simulink model "MPPI"  (R2021b)
settings: Solver=FixedStepAuto  StartTime=0.0  StopTime=10.0  FixedStep=0.01  RelTol=1e-3
undefined symbols (not defined in the file): gaosu, pathdata2
settings Model: Creator=huang.hj  LastModifiedBy=huang.hj

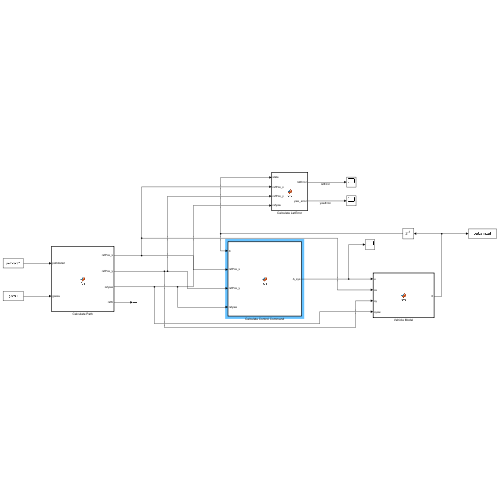
[thumbnail: Simulink's stored preview of the top-level diagram]
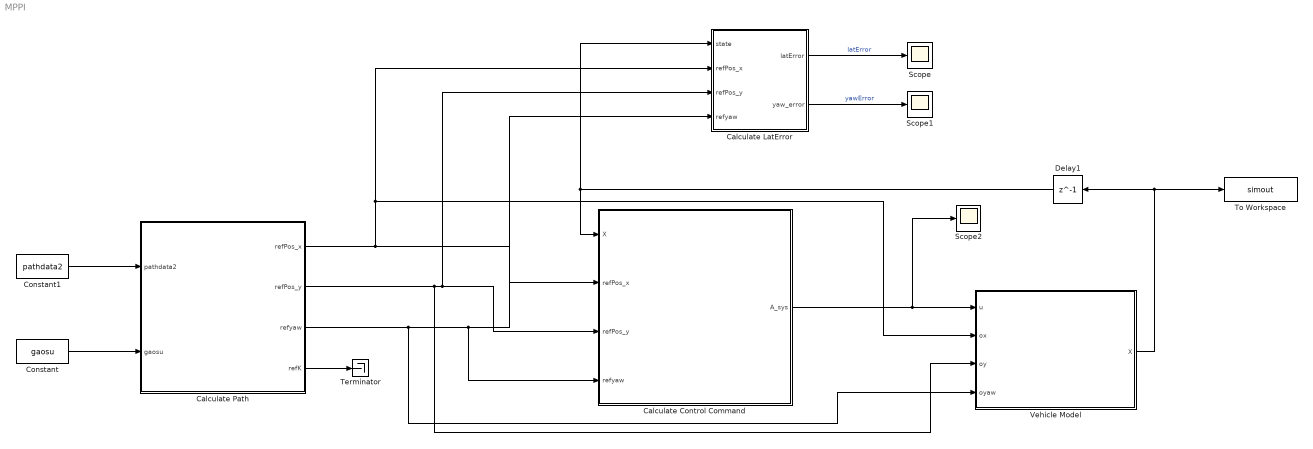
== system MPPI ==
  Calculate Control Command : MATLAB Function  TreatAsAtomicUnit=on
  Calculate LatError : MATLAB Function  TreatAsAtomicUnit=on
  Calculate Path : MATLAB Function  TreatAsAtomicUnit=on
  Constant : Constant  Value=gaosu
  Constant1 : Constant  Value=pathdata2
  Delay1 : Delay  DelayLength=1
  Scope : Scope
  Scope1 : Scope
  Scope2 : Scope
  Terminator : Terminator
  To Workspace : ToWorkspace  VariableName=simout  SaveFormat=Timeseries  SampleTime=-1
  Vehicle Model : MATLAB Function  TreatAsAtomicUnit=on
  wires:
  Constant1/1 -> Calculate Path/1(pathdata2)
  Constant/1 -> Calculate Path/2(gaosu)
  Calculate Path/4(refK) -> Terminator/1
  Calculate Path/3(refyaw) -> Vehicle Model/4(oyaw), Calculate Control Command/4(refyaw), Calculate LatError/4(refyaw)
  Calculate Path/2(refPos_y) -> Vehicle Model/3(oy), Calculate LatError/3(refPos_y), Calculate Control Command/3(refPos_y)
  Calculate Path/1(refPos_x) -> Vehicle Model/2(ox), Calculate LatError/2(refPos_x), Calculate Control Command/2(refPos_x)
  Calculate LatError/1(latError) -> Scope/1  "latError"
  Calculate LatError/2(yaw_error) -> Scope1/1  "yawError"
  Vehicle Model/1(X) -> Delay1/1, To Workspace/1
  Calculate Control Command/1(A_sys) -> Scope2/1, Vehicle Model/1(u)
  Delay1/1 -> Calculate Control Command/1(X), Calculate LatError/1(state)

== matlab function MPPI/Calculate LatError ==
  data: state input; latError output; refPos_x input; refPos_y input; refyaw input; yaw_error output
function [latError, yaw_error] = fcn(state, refPos_x,refPos_y, refyaw)
% persistent step last_latError last_yaw_error
%dt = 0.001;
x = state(1);
y = state(2);
yaw = state(3);
idx = calc_target_index(x,y, refPos_x,refPos_y);


% 求位置、航向角参考量
x_r = refPos_x(idx);
y_r = refPos_y(idx);
heading_r = refyaw(idx); 

% 求位置、航向角的误差
x_error  = x - x_r;
y_error = y - y_r;
yaw_error =  yaw - heading_r;

% 根据百度Apollo，计算横向误差
latError = y_error*cos(heading_r) - x_error*sin(heading_r);

% 将误差值赋值到状态量
% X(1,1) = x_error; 
% X(2,1) = y_error;  
% X(3,1) = yaw_error;

% if isempty(step)
%     latError_rate = 0;
%     yaw_error_rate = 0;
%     last_latError = 0;
%     
%     step = 1;
% else
%     latError_rate = (last_latError-latError)/dt;
%     yaw_error_rate = (last_yaw_error-yaw_error)/dt;
% % end
% last_yaw_error = yaw_error;
% last_latError = latError;
end

== matlab function MPPI/Vehicle Model ==
  data: u input; X output; ox input; oy input; oyaw input
function X = fcn(u,ox,oy,oyaw)
persistent last_state
v = 10;
if isempty(last_state)
    last_state = [ox(1);oy(1);oyaw(1)];
end
dt = 0.01;
L = 4;
xo = last_state(1);
yo = last_state(2);
yaw = last_state(3);
x = xo + v * cos(yaw) * dt;
y = yo + v * sin(yaw) * dt;
yaw = yaw + v / L * tan(u(1)) * dt;
X = [x;y;yaw];
last_state = X;
end

== matlab function MPPI/Calculate Control Command ==
  data: A_sys output; X input; refPos_x input; refPos_y input; refyaw input
function A_sys = fcn(X, refPos_x,refPos_y, refyaw)
persistent last_u u control_a
%% 相关参数定义
K = 200;
N = 50;
param.dt = 0.01;
param.v = 10;              %5m/s
param.m = 1400;
param.g = 9.81;
param.L = 4;


% Variance and Lamda
param.lambda = 10;
param.variance = 1;
param.R = 1;

param.Q = [30 0 0 0;
           0 0 0 0;
           0 0 70 0;
           0 0 0 0];

param.r = 1;
param.omega = 2; %2

filter_param.ts = param.dt;
filter_param.epsilon = 0.78;
filter_param.cutfreq = 4;


% Initialization of input for N time horizone
v = zeros(K,N-1);

% x_cur = zeros(3,N-1);
% u_opt = zeros(1,N-1);
% u_all = zeros(1,N-1,K);
% d_d_u = zeros(1,N-1,K);
if isempty(last_u)
    last_u = 0;
    u = zeros(1,N-1);
    control_a = zeros(1,N-1);
end
a = zeros(K,N-1);
Stk = zeros(1,K);
delta_u = zeros(K,N-1);
delta_limit = deg2rad(30);
d_delta_limit = deg2rad(200);
% Calculating cost for K samples and N finite horizone
for k = 1:K
    x = zeros(3,N);
    x(:,1) = X;
    d_d_u = normrnd(0,param.variance,[1, N-1]);
    %         u_all(:,:,k) = u + d_u;
    for j = 1:N-1
        %d_d_u(j) = clamp_u(d_d_u(j),d_delta_limit,-d_delta_limit);
        delta_u(k,j) = d_d_u(j);
        v(k,j) = u(j)+delta_u(k,j);
        v(k,j) = clamp_u(v(k,j),d_delta_limit,-d_delta_limit);
        %a(k,j) = control_a(j) + v(k,j)*param.dt;
        if j == 1
            a(k,j) = control_a(1) + v(k,j)*param.dt;
        else
            a(k,j) = a(k,j-1) + v(k,j)*param.dt;
        end
        %限制车辆转角极限值
        a(k,j) = clamp_u(a(k,j), delta_limit, -delta_limit);
        x(:,j+1) = vehicle_kinetics(x(:,j) ,a(k,j) ,param);
        [Cost ,~,~] = cost_func(x(:,j+1), a(k,j), refPos_x ,refPos_y ,refyaw ,param);
        Stk(k) = Stk(k) + Cost;
    end
    Stk(k) = Stk(k) + cost_action(a(k,:), last_u, param);
end
for n = 1:N-1
    u(n) = u(n) + totalEntropy(Stk(:) ,delta_u(:,n) ,param);
    control_a(n) = control_a(n) + u(n)*param.dt;
end

if control_a(1) > delta_limit
    A_sys = delta_limit;
elseif control_a(1) < -delta_limit
    A_sys = -delta_limit;
else
    A_sys = control_a(1);
end

A_sys = double_lowpass_filter(A_sys, filter_param);
last_u = A_sys;
u = [u(2:N-1) 0];
%a = [a(2:N-1) 0];
end


function filtered = double_lowpass_filter(unfilter, filter_param)
persistent p_output p_p_output

if isempty(p_output)
    p_output = 0;
    p_p_output = 0;
end

ts = filter_param.ts;
cutoff_freq = filter_param.cutfreq;
epsilon = filter_param.epsilon;

wn = 2*pi*cutoff_freq;

coeff_b1 = -2*exp(-epsilon*wn*ts)*cos(wn*ts*sqrt(1-epsilon^2));
coeff_b2 = exp(-2*wn*epsilon*ts);
coeff_a1 = 1+coeff_b1 + coeff_b2;

filtered = coeff_a1 * unfilter - coeff_b1 * p_output - coeff_b2 * p_p_output;

p_p_output = p_output;
p_output = filtered;
end

function [entropy] = totalEntropy(Sk , del_uk, param)
    % Calculation of expectency over trajectory 
    
    % Normalization of cost function 
%     Sk = Sk./sum(Sk);


    n = length(Sk);
    lambda = param.lambda;
    sum1 = 0;
    sum2 = 0;
    for i = 1:n
        sum1 = sum1 + exp(-(1/lambda)*Sk(i))*del_uk(i);
        sum2 = sum2 + exp(-(1/lambda)*Sk(i));
    end
    if sum2 == 0
        entropy = 0;
    else
        entropy = sum1/sum2;
    end
end

function cost = cost_action(a,a0,param)

omega = param.omega;

cost = (a(1)-a0)*omega*(a(1)-a0);
num = length(a);
for i = 2:num
    cost = cost + (a(i)-a(i-1))*omega*(a(i)-a(i-1));
end
end

function X = vehicle_kinetics(X ,delta ,param)
v = param.v;
dt = param.dt;
L = param.L;
xo = X(1);
yo = X(2);
yaw = X(3);
x = xo + v * cos(yaw) * dt;
y = yo + v * sin(yaw) * dt;
yaw = yaw + v / L * tan(delta) * dt;
X = [x;y;yaw];
end

function result = clamp_u(u, u_max, u_min)
result = u;
if result>u_max
    result = u_max;
end
if result<u_min
    result = u_min;
end
end

function [Cost ,idx,latError] = cost_func(state, u, refPos_x,refPos_y, refyaw, param)
persistent step last_latError last_yaw_error
dt = param.dt;
x = state(1);
y = state(2);
yaw = state(3);
%idx = calc_target_index(x,y, refPos_x,refPos_y);
idx = 1;

% 求位置、航向角参考量
x_r = refPos_x(idx);
y_r = refPos_y(idx);
heading_r = refyaw(idx); 

% 求位置、航向角的误差
x_error  = x - x_r;
y_error = y - y_r;
yaw_error =  yaw - heading_r;

% 根据百度Apollo，计算横向误差
latError = y_error*cos(heading_r) - x_error*sin(heading_r);

% 将误差值赋值到状态量
% X(1,1) = x_error; 
% X(2,1) = y_error;  
% X(3,1) = yaw_error;

if isempty(step)
    latError_rate = 0;
    yaw_error_rate = 0;
    last_latError = 0;
    last_yaw_error = 0;
    step = 1;
else
    latError_rate = (last_latError-latError)/dt;
    yaw_error_rate = (last_yaw_error-yaw_error)/dt;
end
X = zeros(4,1);
X(1,1) = latError; 
X(2,1) = latError_rate;  
X(3,1) = yaw_error;
X(4,1) = yaw_error_rate;
% Q1 = -5.127*exp(-36.37*abs(latError))+5.127*exp(0.7583*abs(latError));
% Q2 = -5.127*exp(-36.37*abs(latError)*dt)+5.127*exp(0.7583*abs(latError)*dt);
% Q3 = -5.127*exp(-36.37*abs(yaw_error))+5.127*exp(0.7583*abs(yaw_error));
% Q4 = -5.127*exp(-36.37*abs(yaw_error_rate*dt))+5.127*exp(0.7583*abs(yaw_error_rate*dt));
% Q = [Q1 0 0 0;
%      0 Q2 0 0;
%      0 0 Q3 0;
%      0 0 0 Q4];
Q = param.Q;

R = param.r;

Cost = X'*Q*X + u*R*u;
last_yaw_error = yaw_error;
last_latError = latError;
end

== matlab function MPPI/Calculate Path ==
  data: refPos_x output; pathdata2 input; gaosu input; refPos_y output; refyaw output; refK output
function [refPos_x, refPos_y, refyaw, refK] = fcn(pathdata2,gaosu)
% persistent refPosx refPosy refPosyaw
% if isempty(refPosyaw)
%% 轨迹处理
switch 1
    case 1
        path = pathdata2(:,1:2);
        path = path(1:1500,:);
    case 2
        path = gaosu(1200:1500,7:8);
    case 3
        %path = path(100:end,:);
end
% path = flip(path);
% 定义参考轨迹
refPos_x = path(:,1);
refPos_y = path(:,2);
% refPos_x = refPos_x(120:225,:);
% refPos_y = refPos_y(120:225,:);
%refPos = [refPos_x, refPos_y];

% 计算航向角和曲率
diff_x = diff(refPos_x) ;
diff_x = [diff_x;diff_x(end)];
diff_y = diff(refPos_y) ;
diff_y = [diff_y;diff_y(end)];
derivative1 = gradient(refPos_y) ./ abs(diff_x);              % 一阶导数
derivative2 = del2(refPos_y) ./ abs(diff_x);                  % 二阶导数
refyaw = atan2(diff_y , diff_x);                   % 航向角
refK = abs(derivative2) ./ (1+derivative1.^2).^(3/2);  % 计算曲率
% refPosx = refPos_x;
% refPosy = refPos_y;
% refPosyaw = refyaw;
% end
% refPos_x = refPosx;
% refPos_y = refPosy;
% refyaw = refPosyaw;
end
